simulink model "Chapter7trial"  (R2017a)
settings: Solver=ode1  StartTime=0.0  StopTime=inf  FixedStep=0.001  RelTol=1e-3  EnableMultiTasking=on
values from neighbouring files (symbols this model uses):
  g = 9.8    [ece486_finalproj1.m]
  Jp = 2.233*10^-4    (= 0.0002233)    [ece486_finalproj1.m]
  Jr = 2.495*10^-5    (= 2.495e-05)    [ece486_finalproj1.m]
  Kup = place(A,B,poles_cl)    [ece486_finalproj1.m]
  lp = 0.1173    [ece486_finalproj1.m]
  lr = 0.1270    (= 0.127)    [ece486_finalproj1.m]
  mp = 0.2164    [ece486_finalproj1.m]
  mr = 0.0850    (= 0.085)    [ece486_finalproj1.m]
libraries: c6xlib x2
Description:
  | Real-Time Van der Pol Simulation
  | 
  | This demonstration shows a real-time version of the Simulink(R) Van der Pol
  | simulation demo. This model does not need any external signals, so it does
  | not need any data acquisition hardware or driver. This makes the model ideal
  | for first experiments with Real-Time Windows Target(TM), without need to
  | worry about proper I/O hardware configuration.
  | 
  | How to run this demo:
  | 
  |   1. Build the model using Tools -> Real-Time Workshop -> Build Model.
  |   2. Connect to the real-time code using Simulation -> Connect to target.
  |   3. Start the real-time execution using Simulation -> Start real-time code.
settings Model: SimulationMode=external  ExtModeTrigDuration=50000  Creator=Houska  LastModifiedBy=lwang114
settings DataIOCC: SaveFormat=Array  SignalLoggingSaveFormat=ModelDataLogs  SignalLoggingName=logsOut
settings OptimizationCC: ExpressionDepthLimit=2147483647  InitFltsAndDblsToZero=on  EfficientMapNaN2IntZero=off
settings DebuggingCC: UnderspecifiedInitializationDetection=Classic  MergeDetectMultiDrivingBlocksExec=none  SignalResolutionControl=TryResolveAllWithWarning  FcnCallInpInsideContextMsg=warning  StateNameClashWarn=warning  SFUnexpectedBacktrackingDiag=warning  SFNoUnconditionalDefaultTransitionDiag=warning  SFExecutionAtInitializationDiag=none
settings ModelReferenceCC: PropagateSignalLabelsOutOfModel=off
settings RTWCC: SystemTargetFile=sldrt.tlc  TemplateMakefile=sldrt.tmf  Description=Simulink Desktop Real-Time  RTWCompilerOptimization=on
settings CodeAppCC: MaxIdLength=95
settings SimulinkDesktopRealTimeCC: TargetPreCompLibLocation=C:\MATLABR2017a\toolbox\sldrt\lib\win64  TargetLangStandard=C89/C90 (ANSI)  SupportVariableSizeSignals=off
settings ConfigComp: CovMetricSettings=dw  CovHtmlReporting=on  CovSaveCumulativeToWorkspaceVar=on  CovSaveSingleToWorkspaceVar=on  CovExternalEMLEnable=off  CovSFcnEnable=off

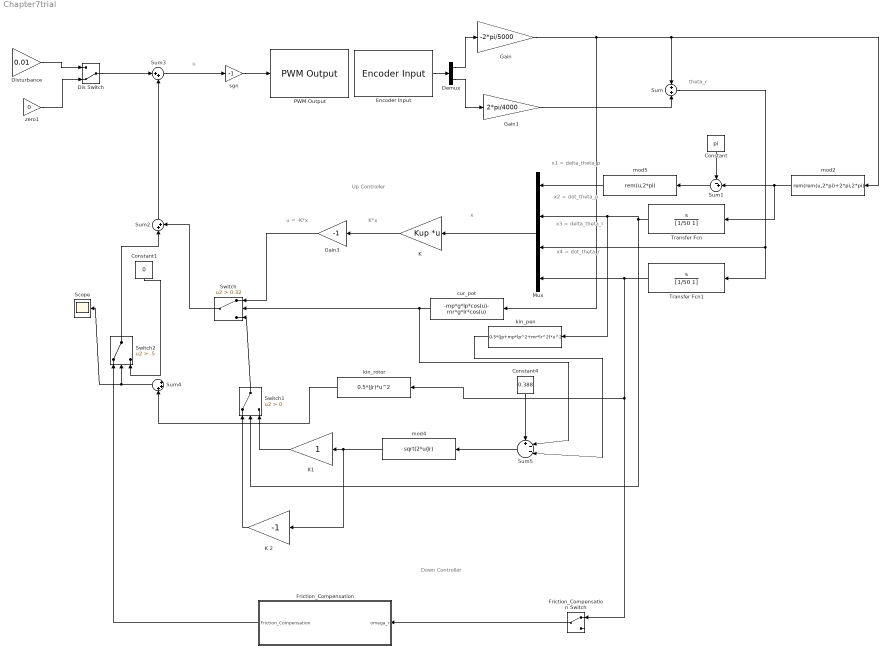
== system Chapter7trial ==
  note: Up Controller
  note: Down Controller
  note: x1 = delta_theta_p
  note: x4 = dot_theta_r
  note: x3 = delta_theta_r
  note: x
  note: u = -K*x
  note: x2 = dot_theta_p
  note: K*x
  note: theta_r
  note: u
  Constant : Constant  Value=pi
  Constant1 : Constant  Value=0
  Constant4 : Constant  Value=0.388
  Demux : Demux  Outputs=2
  Dis Switch : ManualSwitch  CurrentSetting=0
  Disturbance : Gain  Gain=0.01
  Encoder Input : c6xlib/Encoder Input  baseAddr=0x378  channels=[0 1]  sampleTime=str2num(get_param(bdroot, 'FixedStep'))
  Friction_Compensation : Subsystem
  Friction_Compensation Switch : ManualSwitch
  Gain : Gain  Gain=-2*pi/5000
  Gain1 : Gain  Gain=2*pi/4000
  Gain3 : Gain  Gain=-1
  "K " : Gain  Gain=Kup  Multiplication=Matrix(K*u)
  K 2 : Gain  Gain=-1
  K1 : Gain
  Mux : Mux
  PWM Output : c6xlib/PWM Output  baseAddr=0x378  channels=0  initialOutputs=0  finalOutputs=0  sampleTime=str2num(get_param(bdroot, 'FixedStep'))
  Scope : Scope
  Sum : Sum  Inputs=+|+
  Sum1 : Sum  Inputs=-+|
  Sum2 : Sum  Inputs=|++
  Sum3 : Sum  Inputs=|++
  Sum4 : Sum  Inputs=|+++
  Sum5 : Sum  Inputs=+--|
  Switch : Switch  Criteria=u2 > Threshold  Threshold=0.32
  Switch1 : Switch  Criteria=u2 > Threshold
  Switch2 : Switch  Criteria=u2 > Threshold  Threshold=.5
  Transfer Fcn : TransferFcn  Numerator=[1 0]  Denominator=[1/50 1]
  Transfer Fcn1 : TransferFcn  Numerator=[1 0]  Denominator=[1/50 1]
  cur_pot : Fcn  Expr=-mp*g*lp*cos(u)- mr*g*lr*cos(u)
  kin_pen : Fcn  Expr=0.5*(Jp+mp*lp^2+mr*lr^2)*u^2
  kin_rotor : Fcn  Expr=0.5*(Jr)*u^2
  mod2 : Fcn  Expr=rem(rem(u,2*pi)+2*pi,2*pi)
  mod4 : Fcn  Expr=sqrt(2*u/Jr)
  mod5 : Fcn  Expr=rem(u,2*pi)
  sgn : Gain  Gain=-1
  zero1 : Gain  Gain=0
  wires:
  Gain1/1 -> Sum/2
  sgn/1 -> PWM Output/1
  Encoder Input/1 -> Demux/1
  Demux/2 -> Gain1/1
  Transfer Fcn/1 -> Mux/2, kin_pen/1, Switch1/2
  "K "/1 -> Gain3/1
  Demux/1 -> Gain/1
  Constant/1 -> Sum1/1
  Friction_Compensation Switch/1 -> Friction_Compensation/1(omega_r)
  Sum/1 -> Transfer Fcn1/1, Mux/3
  Sum3/1 -> sgn/1
  Sum2/1 -> Sum3/2
  Dis Switch/1 -> Sum3/1
  Disturbance/1 -> Dis Switch/1
  zero1/1 -> Dis Switch/2
  Gain3/1 -> Switch/1
  Mux/1 -> "K "/1
  Transfer Fcn1/1 -> kin_rotor/1, Friction_Compensation Switch/1, Mux/4
  Sum1/1 -> mod5/1
  Gain/1 -> cur_pot/1, mod2/1, Sum/1
  mod2/1 -> Transfer Fcn/1, Sum1/2
  K 2/1 -> Switch1/1
  K1/1 -> Switch1/3
  kin_pen/1 -> Sum5/3
  Constant4/1 -> Sum5/1
  Sum5/1 -> mod4/1
  mod4/1 -> K 2/1, K1/1
  cur_pot/1 -> Switch/2, Sum5/2
  mod5/1 -> Mux/1
  Switch/1 -> Sum2/2
  Switch1/1 -> Switch/3
  Friction_Compensation/1(Friction_Compensation) -> Switch2/1
  kin_rotor/1 -> Sum4/3
  Sum4/1 -> Scope/1, Switch2/2
  Constant1/1 -> Switch2/3
  Switch2/1 -> Sum2/1

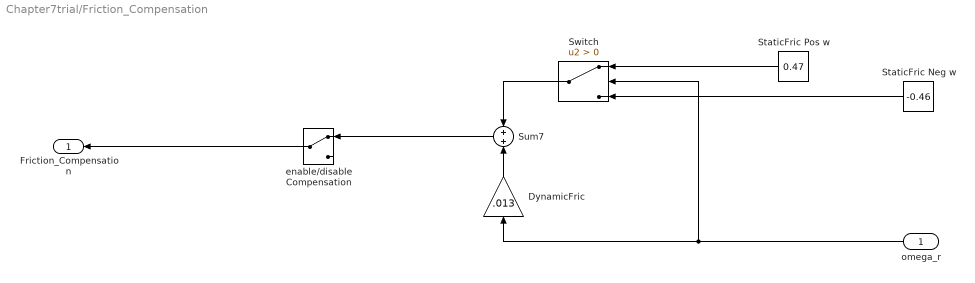
== system Chapter7trial/Friction_Compensation ==
  omega_r : Inport
  DynamicFric : Gain  Gain=.013
  "StaticFric Neg w " : Constant  Value=-0.46
  StaticFric Pos w : Constant  Value=0.47
  Sum7 : Sum
  Switch : Switch  Criteria=u2 > Threshold
  enable/disable Compensation : ManualSwitch
  Friction_Compensation : Outport
  wires:
  "StaticFric Neg w "/1 -> Switch/3
  Sum7/1 -> enable/disable Compensation/1
  omega_r/1 -> Switch/2, DynamicFric/1
  enable/disable Compensation/1 -> Friction_Compensation/1
  Switch/1 -> Sum7/1
  StaticFric Pos w/1 -> Switch/1
  DynamicFric/1 -> Sum7/2
